simulink model "splitPartition"  (R2020a)
settings: Solver=FixedStepDiscrete  StartTime=0.0  StopTime=10.0  RelTol=1e-3
libraries: simulink x1
settings Model: Creator=cyarp  LastModifiedBy=cyarp

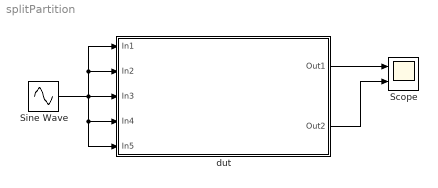
== system splitPartition ==
  Scope : Scope  NumInputPorts=2
  Sine Wave : Sin  SampleTime=0
  dut : Subsystem
  wires:
  Sine Wave/1 -> dut/5(In5), dut/4(In4), dut/3(In3), dut/2(In2), dut/1(In1)
  dut/1(Out1) -> Scope/1
  dut/2(Out2) -> Scope/2

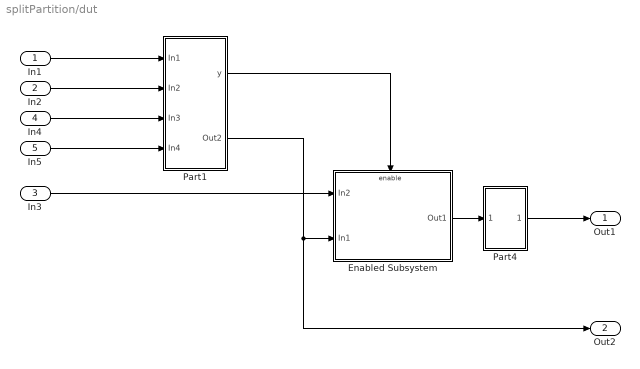
== system splitPartition/dut ==
  In1 : Inport
  In2 : Inport  Port=2
  In3 : Inport  Port=3
  In4 : Inport  Port=4
  In5 : Inport  Port=5
  Enabled Subsystem : Subsystem  TreatAsAtomicUnit=on
  Part1 : Subsystem
  Part4 : Subsystem
  Out1 : Outport
  Out2 : Outport  Port=2
  wires:
  In3/1 -> Enabled Subsystem/1(In2)
  Part1/2(Out2) -> Out2/1, Enabled Subsystem/2(In1)
  In1/1 -> Part1/1(In1)
  In2/1 -> Part1/2(In2)
  In4/1 -> Part1/3(In3)
  In5/1 -> Part1/4(In4)
  Part1/1(y) -> Enabled Subsystem/Enable
  Enabled Subsystem/1(Out1) -> Part4/1(In1)
  Part4/1(Out1) -> Out1/1

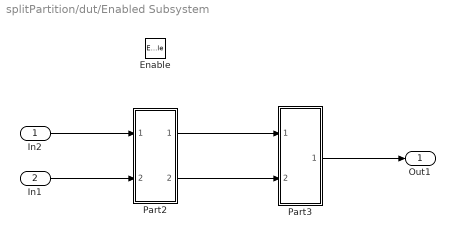
== system splitPartition/dut/Enabled Subsystem ==
  In2 : Inport
  In1 : Inport  Port=2
  Enable : EnablePort
  Part2 : Subsystem
  Part3 : Subsystem
  Out1 : Outport
  wires:
  In2/1 -> Part2/1(In1)
  In1/1 -> Part2/2(In2)
  Part2/1(Out1) -> Part3/1(In1)
  Part2/2(Out2) -> Part3/2(In2)
  Part3/1(Out1) -> Out1/1

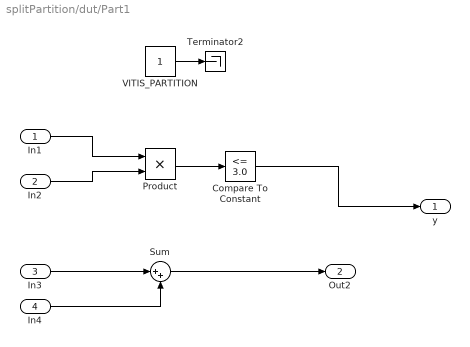
== system splitPartition/dut/Part1 ==
  In1 : Inport
  In2 : Inport  Port=2
  In3 : Inport  Port=3
  In4 : Inport  Port=4
  Compare To Constant : simulink/Logic and Bit Operations/Compare To Constant  relop=<=  const=3.0  OutDataTypeStr=boolean
  Product : Product
  Sum : Sum  Inputs=|++
  Terminator2 : Terminator
  VITIS_PARTITION : Constant
  y : Outport
  Out2 : Outport  Port=2
  wires:
  Compare To Constant/1 -> y/1
  In1/1 -> Product/1
  In4/1 -> Sum/2
  In3/1 -> Sum/1
  In2/1 -> Product/2
  Sum/1 -> Out2/1
  Product/1 -> Compare To Constant/1
  VITIS_PARTITION/1 -> Terminator2/1

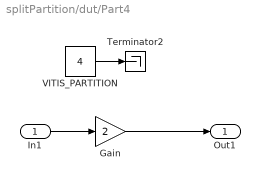
== system splitPartition/dut/Part4 ==
  In1 : Inport
  Gain : Gain  Gain=2
  Terminator2 : Terminator
  VITIS_PARTITION : Constant  Value=4
  Out1 : Outport
  wires:
  In1/1 -> Gain/1
  Gain/1 -> Out1/1
  VITIS_PARTITION/1 -> Terminator2/1

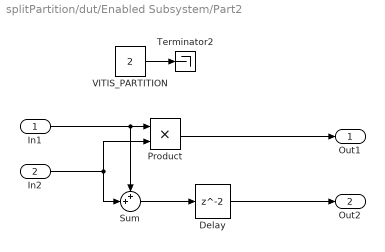
== system splitPartition/dut/Enabled Subsystem/Part2 ==
  In1 : Inport
  In2 : Inport  Port=2
  Delay : Delay
  Product : Product
  Sum : Sum  Inputs=++|
  Terminator2 : Terminator
  VITIS_PARTITION : Constant  Value=2
  Out1 : Outport
  Out2 : Outport  Port=2
  wires:
  Delay/1 -> Out2/1
  Sum/1 -> Delay/1
  Product/1 -> Out1/1
  In2/1 -> Sum/2, Product/2
  In1/1 -> Product/1, Sum/1
  VITIS_PARTITION/1 -> Terminator2/1

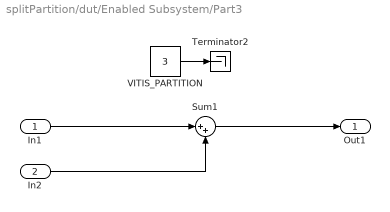
== system splitPartition/dut/Enabled Subsystem/Part3 ==
  In1 : Inport
  In2 : Inport  Port=2
  Sum1 : Sum  Inputs=|++
  Terminator2 : Terminator
  VITIS_PARTITION : Constant  Value=3
  Out1 : Outport
  wires:
  Sum1/1 -> Out1/1
  In2/1 -> Sum1/2
  In1/1 -> Sum1/1
  VITIS_PARTITION/1 -> Terminator2/1
